simulink model "ifft_blocktostream"  (R2023b)
settings: Solver=VariableStepAuto  StartTime=0.0  StopTime=dspb_ifft_multichannel.SimulationTime  RelTol=1e-3
PreLoadFcn:
  | setup_ifft_blocktostream
InitFcn:
  | setup_ifft_blocktostream
StartFcn:
  | setup_ifft_blocktostream
StopFcn:
  | TestAnalysis
values from neighbouring files (symbols this model uses):
  ifft_tb_in = ifft_tb_in_ext    [setup_ifft_blocktostream.m]
undefined symbols (not defined in the file or in its folder): value
libraries: dspsrcs4 x16, DSPBABase x7, DSPBAModelBus x3, lib_lowphy x2, DSPBAPrim x1, simulink x1
settings Model: Creator=5g  LastModifiedBy=5g
settings SolverCC: AlgebraicLoopSolver=TrustRegion
settings DataIOCC: ReturnWorkspaceOutputs=off
settings DebuggingCC: UnconnectedInputMsg=warning  UnconnectedOutputMsg=warning  UnconnectedLineMsg=warning  ArithmeticOperatorsInVariantConditions=warning
settings ModelReferenceCC: EnableRefExpFcnMdlSchedulingChecks=on
settings SFSimCC: CustomCodeUndefinedFunction=UseInterfaceOnly
settings RTWCC: DLArmComputeVersion=19.05

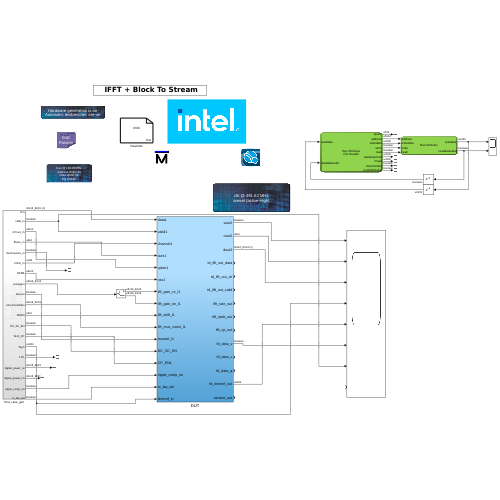
[thumbnail: Simulink's stored preview of the top-level diagram]
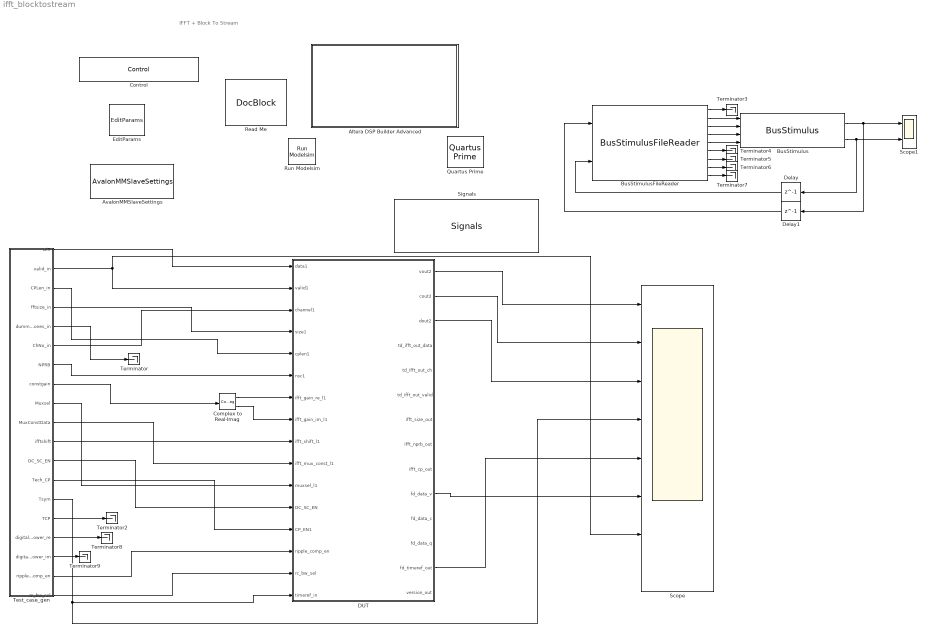
== system ifft_blocktostream ==
  note: IFFT + Block To Stream
  Altera DSP Builder Advanced : Subsystem  mask(DSP Builder Advanced Blockset Ignored Block){}
      settings: OpenFcn=web('http://www.altera.com', '-new');
      mask Display: image(imread('alteralogo.tif'));
  AvalonMMSlaveSettings : DSPBABase/AvalonMMSlaveSettings
  BusStimulus : DSPBAModelBus/BusStimulus  SampleTime=1  version=20140122  hasreaden=on
  BusStimulusFileReader : DSPBAModelBus/BusStimulusFileReader  enabled=on  filename=demo_regs_stimuli.stm  logfilename=demo_regs_stimuli.log  spacewidth=2  addrwidth=14  datawidth=32  SampleTime=-1  version=20140124  hasreaden=on
  Complex to Real-Imag : ComplexToRealImag
  Control : DSPBABase/Control  generate=on  language=VHDL  destination=rtl  make_full_path=off  path_is_relative=on  autotestbench=on  signaldepth=2  coveragetestbench=off  logs=off  spacewidth=2  spacenum=1  addrwidth=10  datawidth=16  dataendian=Big Endian  hierarchicalnames=on  ramThresholdBits=-1  distRamThresholdBits=-1  mlabThresholdBits=-1  hardMultiplierThresholdLuts=-1  version=20090407  errorOnChanMismatch=1  errorOnGPIOMismatch=0  importModelsimResults=0  cycleAccurate=off  reinterpretCastMult=off  paramFile=ifft_blocktostream_params.xml
  DUT : Subsystem
  Delay : Delay  DelayLength=1
  Delay1 : Delay  DelayLength=1
  EditParams : DSPBABase/EditParams  version=20090407
  Quartus Prime : DSPBABase/Quartus Prime  version=20090407
  Read Me : simulink/Model-Wide Utilities/DocBlock  DocumentType=Text
      content=|
      | Model Version : 1.1.1
      | Date of release : 19/10/23
      |
      | Brief description of model :
      |
      | This design includes simulation of low phy components of 5G NR . It consisits of FFT, CP addition
      | Block to stream conversion, Phase compensation, Tx gain scaling.
      |
      | Steps to Run:.
      |
      | 1. Test cases are noted in datagen_testcase_Run.m file.
      | 2. Required testcase can be run to generate test_case_file.mat script.
      |      Automatically, generated vector is given as test input to this .mdl file.
      |      and, Test analysis is run to compare the reference and simulink out data
      |
      | Updates :
      | 1. Digital Power Scaling block  added.
      | 2. wba  delay added based on nprb.
      | 3. PC lut changed from 24bit to 48bit.
      | 4. Workspace log files removed.
      | 5. Masked delay en parameter added
  Run Modelsim : DSPBABase/Run Modelsim  version=20090407
  Scope : Scope  NumInputPorts=8
  Scope1 : Scope  NumInputPorts=2
  Signals : DSPBABase/Signals  clk=clk  freq=240  margin=0  rst=areset  rstactive=High  bus=bus  enbusclock=off  busfreq=491.52  bussync=off  version=20090407
  Terminator{,2..9} (9 alike) : Terminator
  Test_case_gen : Subsystem
  wires:
  Test_case_gen/1(Din) -> DUT/1(data1)
  Test_case_gen/6(ChNo_in) -> DUT/3(channel1)
  Test_case_gen/12(DC_SC_EN) -> DUT/12(DC_SC_EN)
  Test_case_gen/9(Muxsel) -> DUT/11(muxsel_l1)
  Test_case_gen/11(ifftshift) -> DUT/9(ifft_shift_l1)
  Complex to Real-Imag/1 -> DUT/7(ifft_gain_re_l1)
  Test_case_gen/8(constgain) -> Complex to Real-Imag/1
  Complex to Real-Imag/2 -> DUT/8(ifft_gain_im_l1)
  Test_case_gen/2(valid_in) -> DUT/2(valid1), Scope/7
  Test_case_gen/7(NPRB) -> DUT/6(nsc1)
  Test_case_gen/10(MuxConstData) -> DUT/10(ifft_mux_const_l1)
  Test_case_gen/4(fftsize_in) -> DUT/4(size1)
  Test_case_gen/3(CPLen_in) -> DUT/5(cplen1)
  Test_case_gen/13(Tech_CP) -> DUT/13(CP_EN1)
  DUT/1(vout2) -> Scope/1
  DUT/2(cout2) -> Scope/2
  DUT/3(dout2) -> Scope/3
  Test_case_gen/5(dummyones_in) -> Terminator/1
  Test_case_gen/14(Tsym) -> Scope/4, DUT/16(timeref_in)
  Test_case_gen/15(TCP) -> Terminator2/1
  BusStimulusFileReader/6 -> Terminator4/1
  Delay1/1 -> BusStimulusFileReader/1
  Delay/1 -> BusStimulusFileReader/2
  BusStimulusFileReader/3 -> BusStimulus/2
  BusStimulusFileReader/7 -> Terminator5/1
  BusStimulusFileReader/1 -> Terminator3/1
  BusStimulusFileReader/5 -> BusStimulus/4
  BusStimulusFileReader/8 -> Terminator6/1
  BusStimulusFileReader/9 -> Terminator7/1
  BusStimulusFileReader/4 -> BusStimulus/3
  BusStimulus/2 -> Delay/1, Scope1/2
  BusStimulusFileReader/2 -> BusStimulus/1
  BusStimulus/1 -> Delay1/1, Scope1/1
  Test_case_gen/18(ripple_comp_en) -> DUT/14(ripple_comp_en)
  Test_case_gen/19(rc_bw_sel) -> DUT/15(rc_bw_sel)
  Test_case_gen/16(digital_power_re) -> Terminator8/1
  Test_case_gen/17(digital_power_im) -> Terminator9/1
  DUT/13(fd_timeref_out) -> Scope/5
  DUT/10(fd_data_v) -> Scope/6

== system ifft_blocktostream/Altera DSP Builder Advanced ==

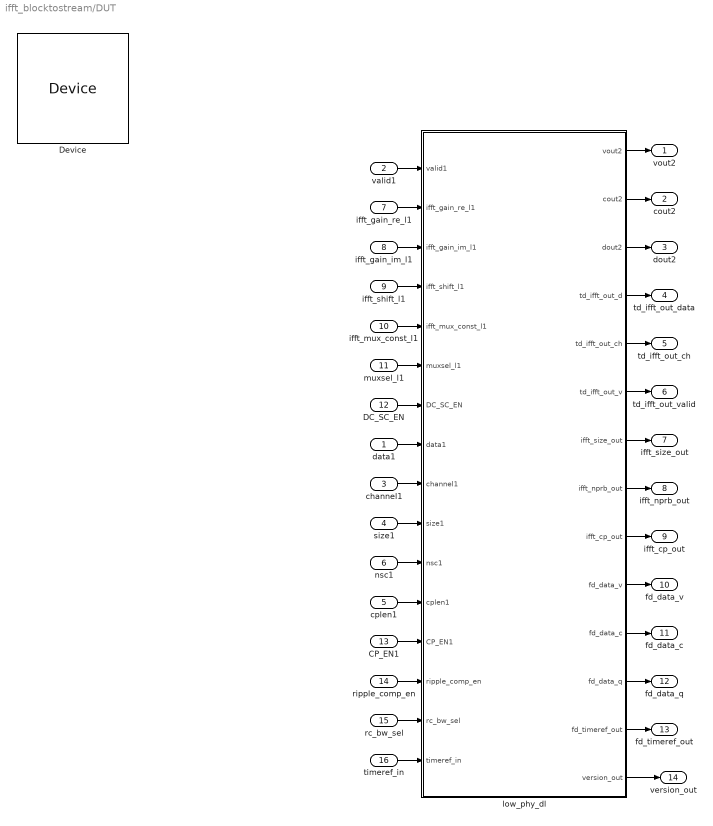
== system ifft_blocktostream/DUT ==
  data1 : Inport
  valid1 : Inport  Port=2
  channel1 : Inport  Port=3
  size1 : Inport  Port=4
  cplen1 : Inport  Port=5
  nsc1 : Inport  Port=6
  ifft_gain_re_l1 : Inport  Port=7
  ifft_gain_im_l1 : Inport  Port=8
  ifft_shift_l1 : Inport  Port=9
  ifft_mux_const_l1 : Inport  Port=10
  muxsel_l1 : Inport  Port=11
  DC_SC_EN : Inport  Port=12
  CP_EN1 : Inport  Port=13
  ripple_comp_en : Inport  Port=14
  rc_bw_sel : Inport  Port=15
  timeref_in : Inport  Port=16
  Device : DSPBABase/Device  family=Cyclone V  deviceMember=Stratix V GX  stratix4device=Stratix IV E  hardcopy4device=HardCopy IV E  stratix5device=Stratix V GX  device=AUTO  speed=6  stratixSpeed=-5  stratix2Speed=-3  stratix3Speed=-3  stratix4gxSpeed=-2  stratix4gtSpeed=-1  cyclone2Speed=-6  cyclone3Speed=-6  arria2Speed=-4  cyclone4eSpeed=-8  stratix5Speed=-3  arria5Speed=-4  arriaSpeed=-6  cyclone3lsSpeed=-7  cyclone5Speed=-6  arria2gzSpeed=-3  nightFurySpeed=-2  ecp2Speed=-7  hardcopycompat=off  version=20140217  max10flashmode=off  max10nomeminit=off
  low_phy_dl : Subsystem
  vout2 : Outport
  cout2 : Outport  Port=2
  dout2 : Outport  Port=3
  td_ifft_out_data : Outport  Port=4
  td_ifft_out_ch : Outport  Port=5
  td_ifft_out_valid : Outport  Port=6
  ifft_size_out : Outport  Port=7
  ifft_nprb_out : Outport  Port=8
  ifft_cp_out : Outport  Port=9
  fd_data_v : Outport  Port=10
  fd_data_c : Outport  Port=11
  fd_data_q : Outport  Port=12
  fd_timeref_out : Outport  Port=13
  version_out : Outport  Port=14
  wires:
  low_phy_dl/11(fd_data_c) -> fd_data_c/1
  low_phy_dl/9(ifft_cp_out) -> ifft_cp_out/1
  low_phy_dl/8(ifft_nprb_out) -> ifft_nprb_out/1
  low_phy_dl/6(td_ifft_out_v) -> td_ifft_out_valid/1
  low_phy_dl/7(ifft_size_out) -> ifft_size_out/1
  low_phy_dl/5(td_ifft_out_ch) -> td_ifft_out_ch/1
  low_phy_dl/4(td_ifft_out_d) -> td_ifft_out_data/1
  low_phy_dl/1(vout2) -> vout2/1
  rc_bw_sel/1 -> low_phy_dl/15(rc_bw_sel)
  low_phy_dl/2(cout2) -> cout2/1
  ripple_comp_en/1 -> low_phy_dl/14(ripple_comp_en)
  valid1/1 -> low_phy_dl/1(valid1)
  low_phy_dl/12(fd_data_q) -> fd_data_q/1
  low_phy_dl/10(fd_data_v) -> fd_data_v/1
  low_phy_dl/3(dout2) -> dout2/1
  data1/1 -> low_phy_dl/8(data1)
  CP_EN1/1 -> low_phy_dl/13(CP_EN1)
  ifft_gain_im_l1/1 -> low_phy_dl/3(ifft_gain_im_l1)
  ifft_mux_const_l1/1 -> low_phy_dl/5(ifft_mux_const_l1)
  muxsel_l1/1 -> low_phy_dl/6(muxsel_l1)
  ifft_gain_re_l1/1 -> low_phy_dl/2(ifft_gain_re_l1)
  ifft_shift_l1/1 -> low_phy_dl/4(ifft_shift_l1)
  cplen1/1 -> low_phy_dl/12(cplen1)
  channel1/1 -> low_phy_dl/9(channel1)
  DC_SC_EN/1 -> low_phy_dl/7(DC_SC_EN)
  nsc1/1 -> low_phy_dl/11(nsc1)
  size1/1 -> low_phy_dl/10(size1)
  timeref_in/1 -> low_phy_dl/16(timeref_in)
  low_phy_dl/13(fd_timeref_out) -> fd_timeref_out/1
  low_phy_dl/14(version_out) -> version_out/1

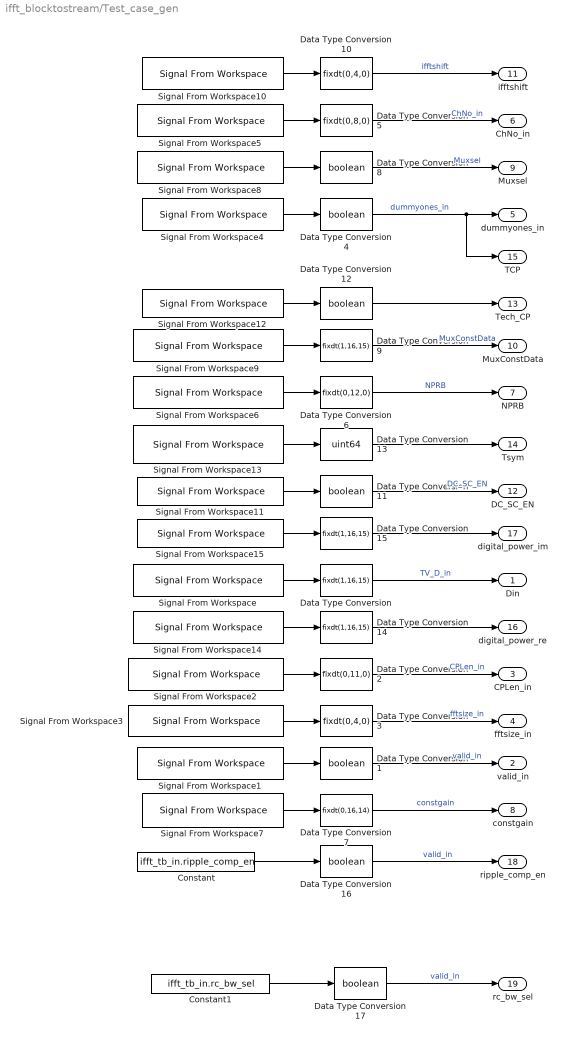
== system ifft_blocktostream/Test_case_gen ==
  Constant : Constant  Value=ifft_tb_in.ripple_comp_en
  Constant1 : Constant  Value=ifft_tb_in.rc_bw_sel
  Data Type Conversion{,9,14..15} (4 alike) : DataTypeConversion  OutDataTypeStr=fixdt(1,16,15)  SaturateOnIntegerOverflow=off  RndMeth=Floor
  Data Type Conversion{1,4,8,11..12,16..17} (7 alike) : DataTypeConversion  OutDataTypeStr=boolean  SaturateOnIntegerOverflow=off  RndMeth=Floor
  Data Type Conversion10 : DataTypeConversion  OutDataTypeStr=fixdt(0,4,0)  SaturateOnIntegerOverflow=off  RndMeth=Floor
  Data Type Conversion13 : DataTypeConversion  OutDataTypeStr=uint64  SaturateOnIntegerOverflow=off  RndMeth=Floor
  Data Type Conversion2 : DataTypeConversion  OutDataTypeStr=fixdt(0,11,0)  SaturateOnIntegerOverflow=off  RndMeth=Floor
  Data Type Conversion3 : DataTypeConversion  OutDataTypeStr=fixdt(0,4,0)  SaturateOnIntegerOverflow=off  RndMeth=Floor
  Data Type Conversion5 : DataTypeConversion  OutDataTypeStr=fixdt(0,8,0)  SaturateOnIntegerOverflow=off  RndMeth=Floor
  Data Type Conversion6 : DataTypeConversion  OutDataTypeStr=fixdt(0,12,0)  SaturateOnIntegerOverflow=off  RndMeth=Floor
  Data Type Conversion7 : DataTypeConversion  OutDataTypeStr=fixdt(0,16,14)  SaturateOnIntegerOverflow=off  RndMeth=Floor
  Signal From Workspace : dspsrcs4/Signal From Workspace  X=ifft_tb_in.d_in  Ts=1  nsamps=1  OutputAfterFinalValue=Cyclic repetition  ignoreOrWarnInputAndFrameLengths=off  OutputFrames=off
  Signal From Workspace1 : dspsrcs4/Signal From Workspace  X=ifft_tb_in.valid_in  Ts=1  nsamps=1  OutputAfterFinalValue=Cyclic repetition  ignoreOrWarnInputAndFrameLengths=off  OutputFrames=off
  Signal From Workspace10 : dspsrcs4/Signal From Workspace  X=ifft_tb_in.ifftshift  Ts=1  nsamps=1  OutputAfterFinalValue=Cyclic repetition  ignoreOrWarnInputAndFrameLengths=off  OutputFrames=off
  Signal From Workspace11 : dspsrcs4/Signal From Workspace  X=ifft_tb_in.DC_SC_EN  Ts=1  nsamps=1  OutputAfterFinalValue=Cyclic repetition  ignoreOrWarnInputAndFrameLengths=off  OutputFrames=off
  Signal From Workspace12 : dspsrcs4/Signal From Workspace  X=ifft_tb_in.Tech_CP  Ts=1  nsamps=1  OutputAfterFinalValue=Cyclic repetition  ignoreOrWarnInputAndFrameLengths=off  OutputFrames=off
  Signal From Workspace13 : dspsrcs4/Signal From Workspace  X=ifft_tb_in.Tsym  Ts=1  nsamps=1  OutputAfterFinalValue=Cyclic repetition  ignoreOrWarnInputAndFrameLengths=off  OutputFrames=off
  Signal From Workspace14 : dspsrcs4/Signal From Workspace  X=ifft_tb_in.Digital_power_real  Ts=1  nsamps=1  OutputAfterFinalValue=Cyclic repetition  ignoreOrWarnInputAndFrameLengths=off  OutputFrames=off
  Signal From Workspace15 : dspsrcs4/Signal From Workspace  X=ifft_tb_in.Digital_power_imag  Ts=1  nsamps=1  OutputAfterFinalValue=Cyclic repetition  ignoreOrWarnInputAndFrameLengths=off  OutputFrames=off
  Signal From Workspace2 : dspsrcs4/Signal From Workspace  X=ifft_tb_in.CPLen_in  Ts=1  nsamps=1  OutputAfterFinalValue=Cyclic repetition  ignoreOrWarnInputAndFrameLengths=off  OutputFrames=off
  Signal From Workspace3 : dspsrcs4/Signal From Workspace  X=ifft_tb_in.fftsize_in  Ts=1  nsamps=1  OutputAfterFinalValue=Cyclic repetition  ignoreOrWarnInputAndFrameLengths=off  OutputFrames=off
  Signal From Workspace4 : dspsrcs4/Signal From Workspace  X=ifft_tb_in.dummyones_in  Ts=1  nsamps=1  OutputAfterFinalValue=Cyclic repetition  ignoreOrWarnInputAndFrameLengths=off  OutputFrames=off
  Signal From Workspace5 : dspsrcs4/Signal From Workspace  X=ifft_tb_in.ChNo_in  Ts=1  nsamps=1  OutputAfterFinalValue=Cyclic repetition  ignoreOrWarnInputAndFrameLengths=off  OutputFrames=off
  Signal From Workspace6 : dspsrcs4/Signal From Workspace  X=ifft_tb_in.NPRB  Ts=1  nsamps=1  OutputAfterFinalValue=Cyclic repetition  ignoreOrWarnInputAndFrameLengths=off  OutputFrames=off
  Signal From Workspace7 : dspsrcs4/Signal From Workspace  X=ifft_tb_in.constgain  Ts=1  nsamps=1  OutputAfterFinalValue=Cyclic repetition  ignoreOrWarnInputAndFrameLengths=off  OutputFrames=off
  Signal From Workspace8 : dspsrcs4/Signal From Workspace  X=ifft_tb_in.Muxsel  Ts=1  nsamps=1  OutputAfterFinalValue=Cyclic repetition  ignoreOrWarnInputAndFrameLengths=off  OutputFrames=off
  Signal From Workspace9 : dspsrcs4/Signal From Workspace  X=ifft_tb_in.MuxConstData  Ts=1  nsamps=1  OutputAfterFinalValue=Cyclic repetition  ignoreOrWarnInputAndFrameLengths=off  OutputFrames=off
  Din : Outport
  valid_in : Outport  Port=2
  CPLen_in : Outport  Port=3
  fftsize_in : Outport  Port=4
  dummyones_in : Outport  Port=5
  ChNo_in : Outport  Port=6
  NPRB : Outport  Port=7
  constgain : Outport  Port=8
  Muxsel : Outport  Port=9
  MuxConstData : Outport  Port=10
  ifftshift : Outport  Port=11
  DC_SC_EN : Outport  Port=12
  Tech_CP : Outport  Port=13
  Tsym : Outport  Port=14
  TCP : Outport  Port=15
  digital_power_re : Outport  Port=16
  digital_power_im : Outport  Port=17
  ripple_comp_en : Outport  Port=18
  rc_bw_sel : Outport  Port=19
  wires:
  Data Type Conversion7/1 -> constgain/1  "constgain"
  Data Type Conversion3/1 -> fftsize_in/1  "fftsize_in"
  Signal From Workspace13/1 -> Data Type Conversion13/1
  Signal From Workspace1/1 -> Data Type Conversion1/1
  Signal From Workspace2/1 -> Data Type Conversion2/1
  Signal From Workspace12/1 -> Data Type Conversion12/1
  Signal From Workspace6/1 -> Data Type Conversion6/1
  Data Type Conversion1/1 -> valid_in/1  "valid_in"
  Signal From Workspace8/1 -> Data Type Conversion8/1
  Data Type Conversion6/1 -> NPRB/1  "NPRB"
  Signal From Workspace14/1 -> Data Type Conversion14/1
  Data Type Conversion5/1 -> ChNo_in/1  "ChNo_in"
  Signal From Workspace11/1 -> Data Type Conversion11/1
  Signal From Workspace4/1 -> Data Type Conversion4/1
  Signal From Workspace3/1 -> Data Type Conversion3/1
  Signal From Workspace/1 -> Data Type Conversion/1
  Signal From Workspace9/1 -> Data Type Conversion9/1
  Signal From Workspace5/1 -> Data Type Conversion5/1
  Signal From Workspace7/1 -> Data Type Conversion7/1
  Data Type Conversion11/1 -> DC_SC_EN/1  "DC_SC_EN"
  Data Type Conversion8/1 -> Muxsel/1  "Muxsel"
  Data Type Conversion10/1 -> ifftshift/1  "ifftshift"
  Data Type Conversion4/1 -> TCP/1, dummyones_in/1  "dummyones_in"
  Data Type Conversion/1 -> Din/1  "TV_D_in"
  Data Type Conversion12/1 -> Tech_CP/1
  Data Type Conversion9/1 -> MuxConstData/1  "MuxConstData"
  Data Type Conversion13/1 -> Tsym/1
  Data Type Conversion15/1 -> digital_power_im/1
  Signal From Workspace15/1 -> Data Type Conversion15/1
  Data Type Conversion14/1 -> digital_power_re/1
  Signal From Workspace10/1 -> Data Type Conversion10/1
  Data Type Conversion2/1 -> CPLen_in/1  "CPLen_in"
  Constant/1 -> Data Type Conversion16/1
  Constant1/1 -> Data Type Conversion17/1
  Data Type Conversion16/1 -> ripple_comp_en/1  "valid_in"
  Data Type Conversion17/1 -> rc_bw_sel/1  "valid_in"

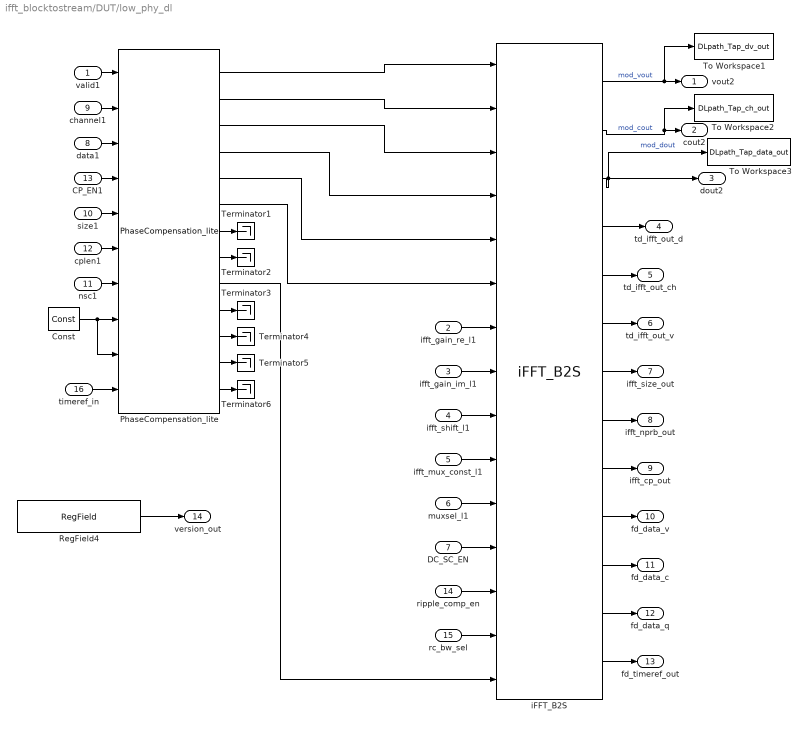
== system ifft_blocktostream/DUT/low_phy_dl ==
  valid1 : Inport
  ifft_gain_re_l1 : Inport  Port=2
  ifft_gain_im_l1 : Inport  Port=3
  ifft_shift_l1 : Inport  Port=4
  ifft_mux_const_l1 : Inport  Port=5
  muxsel_l1 : Inport  Port=6
  DC_SC_EN : Inport  Port=7
  data1 : Inport  Port=8
  channel1 : Inport  Port=9
  size1 : Inport  Port=10
  nsc1 : Inport  Port=11
  cplen1 : Inport  Port=12
  CP_EN1 : Inport  Port=13
  ripple_comp_en : Inport  Port=14
  rc_bw_sel : Inport  Port=15
  timeref_in : Inport  Port=16
  Const : DSPBAPrim/Const  primtype=const  nInputs=0  nOutputs=1  omode=boolean  otype=fixdt(0,3,0)  scale=0  rndmethod=Unbiased  factor=1  satmethod=Symmetric  shift_vec=[0 1 2 -1]  value=0  inPortNames=['+'; '+';]  outPortNames=[' ']  dspbaimage=dspba_prim.svg  text=fprintf('%s', num2str(value));  style=Optimised  visibilities=8 + 1024 + 2^18 + 2^20  floatPrecision=float32_m23  warnSaturation=on  version=20211007  SampleTime=inf
  PhaseCompensation_lite : lib_lowphy/PhaseCompensation_lite  Tc=1/122.88e6  CP_1=352  CP_2=288  PhaseGen_TXRX=1  Op_frac_scaling=2^-14  reg_mem_offset_rf_freq=0  reg_mem_offset_Phase_comp_enable=1  reg_mem_offset_tx_rx_sel=2
      link override ComplexMixer/ComplexMixer: latency=5
      link override PhasorGenerate/ChannelOut: latency=36
      link override SOP_EOP_gen/channel_RXG1_out: latency=0
  RegField4 : DSPBAModelBus/RegField  reg_name=reg_mem_offset_version  reg_rwmode=Read/Write  reg_msb=31  reg_lsb=0  reg_mode=Specify via dialog  reg_type=ufix(32)  reg_scale=2^0  reg_init=Version_reg_val  reg_desc=version_out  reg_modal=off  reg_desc0=0  reg_desc1=0  reg_desc2=0  reg_desc3=0  reg_desc4=0  reg_desc5=0  reg_desc6=0  reg_desc7=0  reg_addr=3  SampleTime=-1  version=20090407
  Terminator{1..6} (6 alike) : Terminator
  To Workspace1 : ToWorkspace  VariableName=DLpath_Tap_dv_out  SaveFormat=Timeseries  SampleTime=-1
  To Workspace2 : ToWorkspace  VariableName=DLpath_Tap_ch_out  SaveFormat=Timeseries  SampleTime=-1
  To Workspace3 : ToWorkspace  VariableName=DLpath_Tap_data_out  SaveFormat=Timeseries  SampleTime=-1
  iFFT_B2S : lib_lowphy/iFFT_B2S  iFFTmaxsize=12  iFFTminsize=9  iFFTstages=12  Tx_scaling=2^-14  Bw_Delay_en=1  rc_out_frac=13
      link override B2S/B2S_Inst/CB/SampleReggen/SampleregMaxval_Calc2/d: augmented=7
      link override B2S/B2S_Inst/CB/SampleReggen/SampleregMaxval_Calc2/d1: augmented=7
      link override B2S/B2S_Inst/CB/Valid1: augmented=7
      link override B2S/B2S_Inst/GPOut: latency=5
      link override IFFT/Input_signal_latch/ChannelIn: dataSignals=11
      link override IFFT/Input_signal_latch/ChannelOut: dataSignals=11
      link override IFFT/VIFFT/BRandSCMap/ChannelIn: dataSignals=8
      link override IFFT/VIFFT/BRandSCMap/ChannelOut: latency=16  dataSignals=6
      link override IFFT/VIFFT/TXGainComp/ChannelOut: latency=9
      link override IFFT/VIFFT/VFFT/ChannelOut1: latency=56
  vout2 : Outport
  cout2 : Outport  Port=2
  dout2 : Outport  Port=3
  td_ifft_out_d : Outport  Port=4
  td_ifft_out_ch : Outport  Port=5
  td_ifft_out_v : Outport  Port=6
  ifft_size_out : Outport  Port=7
  ifft_nprb_out : Outport  Port=8
  ifft_cp_out : Outport  Port=9
  fd_data_v : Outport  Port=10
  fd_data_c : Outport  Port=11
  fd_data_q : Outport  Port=12
  fd_timeref_out : Outport  Port=13
  version_out : Outport  Port=14
  wires:
  iFFT_B2S/8 -> ifft_nprb_out/1
  RegField4/1 -> version_out/1
  valid1/1 -> PhaseCompensation_lite/1
  iFFT_B2S/2 -> cout2/1, To Workspace2/1  "mod_cout"
  PhaseCompensation_lite/4 -> iFFT_B2S/4
  CP_EN1/1 -> PhaseCompensation_lite/4
  PhaseCompensation_lite/1 -> iFFT_B2S/1
  ifft_mux_const_l1/1 -> iFFT_B2S/10
  cplen1/1 -> PhaseCompensation_lite/6
  PhaseCompensation_lite/2 -> iFFT_B2S/2
  Const/1 -> PhaseCompensation_lite/9, PhaseCompensation_lite/8
  PhaseCompensation_lite/5 -> iFFT_B2S/5
  size1/1 -> PhaseCompensation_lite/5
  data1/1 -> PhaseCompensation_lite/3
  PhaseCompensation_lite/7 -> Terminator1/1
  nsc1/1 -> PhaseCompensation_lite/7
  ifft_gain_im_l1/1 -> iFFT_B2S/8
  iFFT_B2S/7 -> ifft_size_out/1
  ifft_gain_re_l1/1 -> iFFT_B2S/7
  rc_bw_sel/1 -> iFFT_B2S/14
  ifft_shift_l1/1 -> iFFT_B2S/9
  channel1/1 -> PhaseCompensation_lite/2
  DC_SC_EN/1 -> iFFT_B2S/12
  muxsel_l1/1 -> iFFT_B2S/11
  ripple_comp_en/1 -> iFFT_B2S/13
  iFFT_B2S/1 -> To Workspace1/1, vout2/1  "mod_vout"
  PhaseCompensation_lite/3 -> iFFT_B2S/3
  iFFT_B2S/3 -> dout2/1, To Workspace3/1  "mod_dout"
  iFFT_B2S/9 -> ifft_cp_out/1
  PhaseCompensation_lite/6 -> iFFT_B2S/6
  iFFT_B2S/4 -> td_ifft_out_d/1
  iFFT_B2S/6 -> td_ifft_out_v/1
  iFFT_B2S/5 -> td_ifft_out_ch/1
  PhaseCompensation_lite/8 -> Terminator2/1
  PhaseCompensation_lite/10 -> Terminator3/1
  PhaseCompensation_lite/11 -> Terminator4/1
  PhaseCompensation_lite/12 -> Terminator5/1
  PhaseCompensation_lite/13 -> Terminator6/1
  timeref_in/1 -> PhaseCompensation_lite/10
  iFFT_B2S/10 -> fd_data_v/1
  iFFT_B2S/11 -> fd_data_c/1
  iFFT_B2S/12 -> fd_data_q/1
  iFFT_B2S/13 -> fd_timeref_out/1
  PhaseCompensation_lite/9 -> iFFT_B2S/15
